simulink model "PA_Reactor_2019"  (R2018b)
settings: Solver=ode15s  StartTime=0  StopTime=400  RelTol=1e-3
libraries: simulink x13
settings Model: Creator=fmala  LastModifiedBy=andreas
settings OptimizationCC: EfficientMapNaN2IntZero=off
settings HardwareCC: TargetBitPerLong=64  TargetBitPerPointer=64  TargetBitPerSizeT=64  TargetBitPerPtrDiffT=64  TargetLongLongMode=on  TargetIntDivRoundTo=Zero  TargetEndianess=LittleEndian  TargetWordSize=64  TargetHWDeviceType=MATLAB Host  ProdEqTarget=off
settings CodeAppCC: MaxIdLength=128
settings GRTTargetCC: TargetLangStandard=C89/C90 (ANSI)  CombineOutputUpdateFcns=off  GRTInterface=on

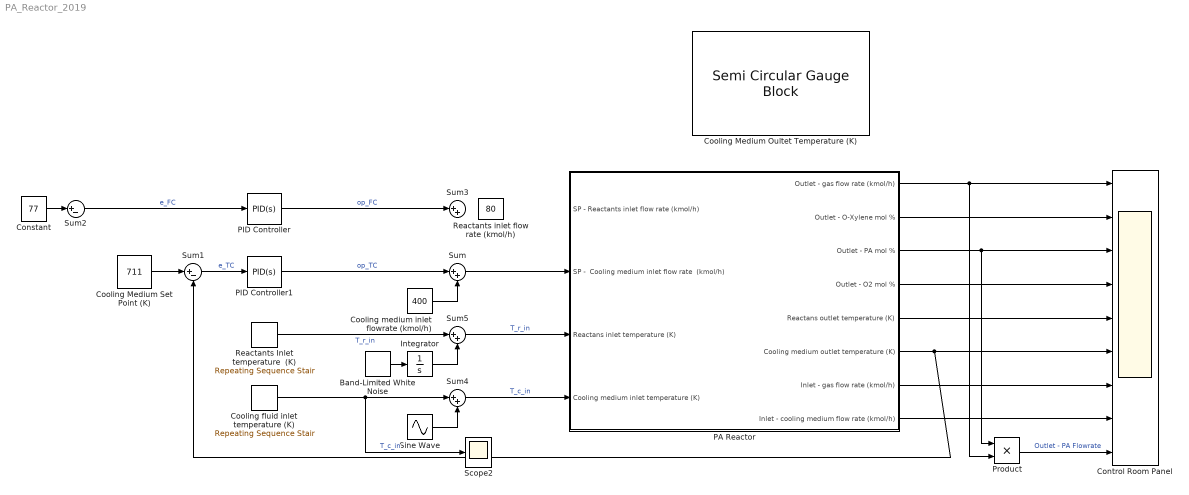
== system PA_Reactor_2019 ==
  Band-Limited White Noise : simulink/Sources/Band-Limited White Noise  Cov=1  Ts=1  seed=[23341]
  Constant : Constant  Value=77
  Control Room Panel : Scope  NumInputPorts=9
  Cooling Medium Oultet Temperature (K) : SemiCircularGaugeBlock  WebBlockId=63  ScaleMin=680  ScaleMax=780
  "Cooling Medium Set Point (K) " : Constant  Value=711  VectorParams1D=off  SampleTime=-1
  Cooling fluid inlet temperature (K) : simulink/Sources/Repeating Sequence Stair  OutValues=[680 680 685 690 695 705 705 705 705 705].'  tsamp=30  OutMin=[]  OutMax=[]  OutDataTypeStr=double  OutputDataTypeScalingMode=double  OutDataType=fixdt(0,8)  ConRadixGroup=Best Precision: Vector-wise  OutScaling=2^-12
  Cooling medium inlet flowrate (kmol/h) : Constant  Value=400
  Integrator : Integrator
  PA Reactor : Subsystem
  PID Controller : simulink/Continuous/PID Controller  Controller=PID  Form=Parallel  TimeDomain=Continuous-time  SampleTime=-1  IntegratorMethod=Forward Euler  FilterMethod=Forward Euler  ControllerParametersSource=internal  P=-0.2  I=0  D=0  UseFilter=on  N=100  TunerSelectOption=Transfer Function Based (PID Tuner App)  InitialConditionSource=internal  InitialConditionForIntegrator=0  InitialConditionForFilter=0  DifferentiatorICPrevScaledInput=0  ExternalReset=none  TrackingMode=off  Kt=1  LimitOutput=off  UpperSaturationLimit=inf  LowerSaturationLimit=-inf  LinearizeAsGain=on  AntiWindupMode=none  Kb=1  POutMin=[]  POutMax=[]  IOutMin=[]  IOutMax=[]  DOutMin=[]  DOutMax=[]  NOutMin=[]  NOutMax=[]  SumOutMin=[]  SumOutMax=[]  SaturationOutMin=[]  SaturationOutMax=[]  PParamMin=[]  PParamMax=[]  IParamMin=[]  IParamMax=[]  DParamMin=[]  DParamMax=[]  NParamMin=[]  NParamMax=[]  KbParamMin=[]  KbParamMax=[]  KtParamMin=[]  KtParamMax=[]  KbOutMin=[]  KbOutMax=[]  KtOutMin=[]  KtOutMax=[]  IntegratorOutMin=[]  IntegratorOutMax=[]  FilterOutMin=[]  FilterOutMax=[]  SumI1OutMin=[]  SumI1OutMax=[]  SumI2OutMin=[]  SumI2OutMax=[]  SumI3OutMin=[]  SumI3OutMax=[]  SumI4OutMin=[]  SumI4OutMax=[]  SumDOutMin=[]  SumDOutMax=[]  DifferentiatorOutMin=[]  DifferentiatorOutMax=[]  FilterDiffOutCoefMin=[]  FilterDiffOutCoefMax=[]  ReciprocalOutMin=[]  ReciprocalOutMax=[]  SumDenOutMin=[]  SumDenOutMax=[]  SumNumOutMin=[]  SumNumOutMax=[]  DivideOutMin=[]  DivideOutMax=[]  IntegratorContinuousStateAttributes=''  IntegratorStateMustResolveToSignalObject=off  IntegratorRTWStateStorageClass=Auto  FilterContinuousStateAttributes=''  FilterStateMustResolveToSignalObject=off  FilterRTWStateStorageClass=Auto  ParallelPVariant=InternalParameters  IdealPVariant=Disabled  IVariant=InternalParameters  DVariant=InternalParameters  IntegratorVariant=Continuous  SatVariant=Disabled  AWVariant=Passthrough  PCopyVariant=Disabled  TRVariant=Disabled  FdbkBlocksVariant=Forward  IdealPFdbkVariant=Disabled  SatFdbkVariant=Disabled  DerivativeFilterVariant=ContFilter  NVariant=InternalParameters  NCopyVariant=Disabled  FilterICVariant=InternalICsFilter  IntegratorICVariant=InternalICs  ExternalResetVariant=Disabled  TRSumVariant=Passthrough  SumFdbkVariant=Disabled  SumVariant=Sum_PID
  PID Controller1 : simulink/Continuous/PID Controller  Controller=PID  Form=Ideal  TimeDomain=Continuous-time  SampleTime=-1  IntegratorMethod=Forward Euler  FilterMethod=Forward Euler  ControllerParametersSource=internal  P=-3  I=2  D=0  UseFilter=on  N=100  TunerSelectOption=Transfer Function Based (PID Tuner App)  InitialConditionSource=internal  InitialConditionForIntegrator=0  InitialConditionForFilter=0  DifferentiatorICPrevScaledInput=0  ExternalReset=none  TrackingMode=off  Kt=1  LimitOutput=off  UpperSaturationLimit=inf  LowerSaturationLimit=-inf  LinearizeAsGain=on  AntiWindupMode=none  Kb=1  POutMin=[]  POutMax=[]  IOutMin=[]  IOutMax=[]  DOutMin=[]  DOutMax=[]  NOutMin=[]  NOutMax=[]  SumOutMin=[]  SumOutMax=[]  SaturationOutMin=[]  SaturationOutMax=[]  PParamMin=[]  PParamMax=[]  IParamMin=[]  IParamMax=[]  DParamMin=[]  DParamMax=[]  NParamMin=[]  NParamMax=[]  KbParamMin=[]  KbParamMax=[]  KtParamMin=[]  KtParamMax=[]  KbOutMin=[]  KbOutMax=[]  KtOutMin=[]  KtOutMax=[]  IntegratorOutMin=[]  IntegratorOutMax=[]  FilterOutMin=[]  FilterOutMax=[]  SumI1OutMin=[]  SumI1OutMax=[]  SumI2OutMin=[]  SumI2OutMax=[]  SumI3OutMin=[]  SumI3OutMax=[]  SumI4OutMin=[]  SumI4OutMax=[]  SumDOutMin=[]  SumDOutMax=[]  DifferentiatorOutMin=[]  DifferentiatorOutMax=[]  FilterDiffOutCoefMin=[]  FilterDiffOutCoefMax=[]  ReciprocalOutMin=[]  ReciprocalOutMax=[]  SumDenOutMin=[]  SumDenOutMax=[]  SumNumOutMin=[]  SumNumOutMax=[]  DivideOutMin=[]  DivideOutMax=[]  IntegratorContinuousStateAttributes=''  IntegratorStateMustResolveToSignalObject=off  IntegratorRTWStateStorageClass=Auto  FilterContinuousStateAttributes=''  FilterStateMustResolveToSignalObject=off  FilterRTWStateStorageClass=Auto  ParallelPVariant=Passthrough  IdealPVariant=InternalParameters  IVariant=InternalParameters  DVariant=InternalParameters  IntegratorVariant=Continuous  SatVariant=Disabled  AWVariant=Passthrough  PCopyVariant=Disabled  TRVariant=Disabled  FdbkBlocksVariant=Forward  IdealPFdbkVariant=Disabled  SatFdbkVariant=Disabled  DerivativeFilterVariant=ContFilter  NVariant=InternalParameters  NCopyVariant=Disabled  FilterICVariant=InternalICsFilter  IntegratorICVariant=InternalICs  ExternalResetVariant=Disabled  TRSumVariant=Passthrough  SumFdbkVariant=Disabled  SumVariant=Sum_PID
  Product : Product
  Reactants Inlet temperature  (K) : simulink/Sources/Repeating Sequence Stair  OutValues=[690].'  tsamp=10  OutMin=[]  OutMax=[]  OutDataTypeStr=double  OutputDataTypeScalingMode=double  OutDataType=fixdt(0,8)  ConRadixGroup=Best Precision: Vector-wise  OutScaling=2^-12
  "Reactants inlet flow rate (kmol/h) " : Constant  Value=80
  Scope2 : Scope
  Sine Wave : Sin  Amplitude=20  Frequency=pi/200  SampleTime=0
  Sum{,3..5} (4 alike) : Sum  Inputs=|++
  Sum1 : Sum  Inputs=|+-
  Sum2 : Sum  Inputs=|+-
  wires:
  PA Reactor/1(Outlet - gas flow rate (kmol/h)) -> Control Room Panel/1, Product/2
  PA Reactor/2(Outlet - O-Xylene mol %) -> Control Room Panel/2
  PA Reactor/3(Outlet - PA mol %) -> Control Room Panel/3, Product/1
  PA Reactor/4(Outlet - O2 mol %) -> Control Room Panel/4
  PA Reactor/7(Inlet - gas flow rate (kmol/h)) -> Control Room Panel/7
  PA Reactor/8(Inlet - cooling medium flow rate (kmol/h)) -> Control Room Panel/8
  PA Reactor/6(Cooling medium outlet temperature (K)) -> Sum1/2, Control Room Panel/6
  Cooling fluid inlet temperature (K)/1 -> Sum4/1, Scope2/1  "T_c_in"
  Sum1/1 -> PID Controller1/1  "e_TC"
  PID Controller1/1 -> Sum/1  "op_TC"
  PA Reactor/5(Reactans outlet temperature (K)) -> Control Room Panel/5
  Constant/1 -> Sum2/1
  Sum2/1 -> PID Controller/1  "e_FC"
  PID Controller/1 -> Sum3/1  "op_FC"
  Cooling medium inlet flowrate (kmol/h)/1 -> Sum/2
  Sum/1 -> PA Reactor/2(SP -  Cooling medium inlet flow rate  (kmol/h))
  "Cooling Medium Set Point (K) "/1 -> Sum1/1
  Sum4/1 -> PA Reactor/4(Cooling medium inlet temperature (K))  "T_c_in"
  Sine Wave/1 -> Sum4/2
  Reactants Inlet temperature  (K)/1 -> Sum5/1  "T_r_in"
  Sum5/1 -> PA Reactor/3(Reactans inlet temperature (K))  "T_r_in"
  Integrator/1 -> Sum5/2
  Band-Limited White Noise/1 -> Integrator/1
  Product/1 -> Control Room Panel/9  "Outlet - PA Flowrate"

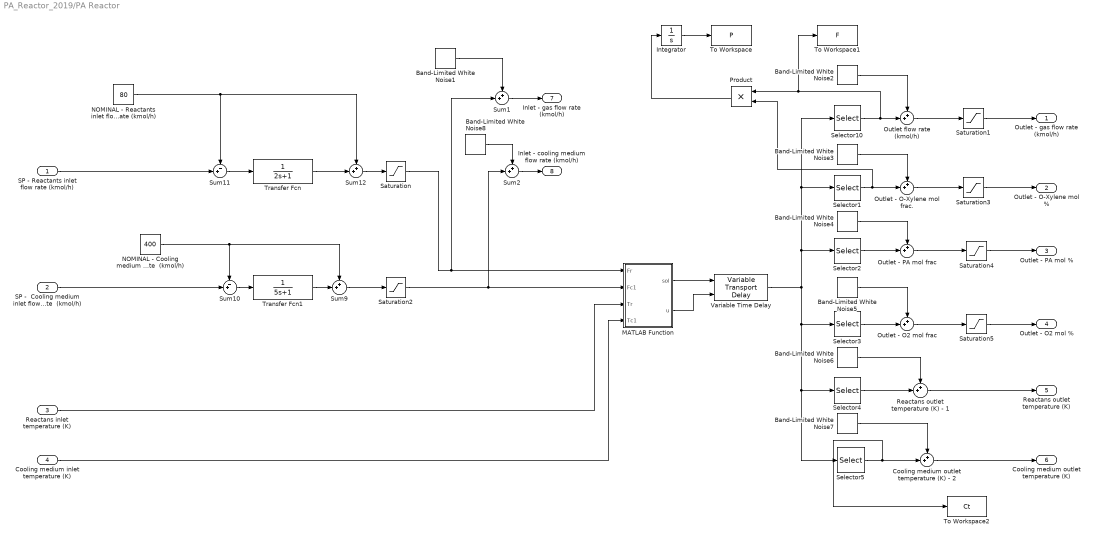
== system PA_Reactor_2019/PA Reactor ==
  SP - Reactants inlet flow rate (kmol/h) : Inport
  SP -  Cooling medium inlet flow rate  (kmol/h) : Inport  Port=2
  Reactans inlet temperature (K) : Inport  Port=3
  Cooling medium inlet temperature (K) : Inport  Port=4
  Band-Limited White Noise1 : simulink/Sources/Band-Limited White Noise  Cov=[0.001]  Ts=0.01  seed=[1111]
  Band-Limited White Noise2 : simulink/Sources/Band-Limited White Noise  Cov=[0.001]  Ts=0.01  seed=[1]
  Band-Limited White Noise3 : simulink/Sources/Band-Limited White Noise  Cov=[0.0001]  Ts=0.5  seed=[3341]
  Band-Limited White Noise4 : simulink/Sources/Band-Limited White Noise  Cov=[0.0001]  Ts=0.5  seed=[2355341]
  Band-Limited White Noise5 : simulink/Sources/Band-Limited White Noise  Cov=[0.0001]  Ts=0.5  seed=[7341]
  Band-Limited White Noise6 : simulink/Sources/Band-Limited White Noise  Cov=[0.002]  Ts=0.01  seed=[241]
  Band-Limited White Noise7 : simulink/Sources/Band-Limited White Noise  Cov=[0.008]  Ts=0.03  seed=[23341]
  Band-Limited White Noise8 : simulink/Sources/Band-Limited White Noise  Cov=[0.001]  Ts=0.01  seed=[1575777]
  Cooling medium outlet temperature (K) - 2 : Sum  Inputs=++|
  Integrator : Integrator
  MATLAB Function : MATLAB Function  TreatAsAtomicUnit=on
  NOMINAL - Cooling medium inlet flow rate  (kmol/h) : Constant  Value=400
  NOMINAL - Reactants inlet flow rate (kmol/h) : Constant  Value=80
  Outlet - O-Xylene mol frac. : Sum  Inputs=++|
  Outlet - O2 mol frac : Sum  Inputs=++|
  Outlet - PA mol frac : Sum  Inputs=++|
  Outlet flow rate (kmol/h) : Sum  Inputs=++|
  Product : Product
  Reactans outlet temperature (K) - 1 : Sum  Inputs=++|
  Saturation : Saturate  UpperLimit=250  LowerLimit=10
  Saturation1 : Saturate  UpperLimit=500  LowerLimit=0
  Saturation2 : Saturate  UpperLimit=1000  LowerLimit=100
  Saturation3 : Saturate  UpperLimit=100  LowerLimit=0
  Saturation4 : Saturate  UpperLimit=100  LowerLimit=0
  Saturation5 : Saturate  UpperLimit=100  LowerLimit=0
  Selector1 : Selector  InputPortWidth=6  IndexOptions=Index vector (dialog)  Indices=[2]  OutputSizes=1
  Selector10 : Selector  InputPortWidth=6  IndexOptions=Index vector (dialog)  Indices=[1]  OutputSizes=1
  Selector2 : Selector  InputPortWidth=6  IndexOptions=Index vector (dialog)  Indices=[3]  OutputSizes=1
  Selector3 : Selector  InputPortWidth=6  IndexOptions=Index vector (dialog)  Indices=[4]  OutputSizes=1
  Selector4 : Selector  InputPortWidth=6  IndexOptions=Index vector (dialog)  Indices=[5]  OutputSizes=1
  Selector5 : Selector  InputPortWidth=6  IndexOptions=Index vector (dialog)  Indices=[6]  OutputSizes=1
  Sum{1..2,9,12} (4 alike) : Sum  Inputs=++|
  Sum10 : Sum  Inputs=-+|
  Sum11 : Sum  Inputs=-+|
  To Workspace : ToWorkspace  VariableName=P  SaveFormat=Timeseries  SampleTime=-1
  To Workspace1 : ToWorkspace  VariableName=F  SaveFormat=Timeseries  SampleTime=-1
  To Workspace2 : ToWorkspace  VariableName=Ct  SaveFormat=Timeseries  SampleTime=-1
  Transfer Fcn : TransferFcn  Denominator=[2 1]
  Transfer Fcn1 : TransferFcn  Denominator=[5 1]
  Variable Time Delay : VariableTransportDelay  MaximumDelay=25  InitialOutput=[90.36 0 0.85 2.12 711 711]  MaximumPoints=3072  ZeroDelay=on
  Outlet - gas flow rate (kmol/h) : Outport
  Outlet - O-Xylene mol % : Outport  Port=2
  Outlet - PA mol % : Outport  Port=3
  Outlet - O2 mol % : Outport  Port=4
  Reactans outlet temperature (K) : Outport  Port=5
  Cooling medium outlet temperature (K) : Outport  Port=6
  Inlet - gas flow rate (kmol/h) : Outport  Port=7
  Inlet - cooling medium flow rate (kmol/h) : Outport  Port=8
  wires:
  Selector3/1 -> Outlet - O2 mol frac/2
  Variable Time Delay/1 -> Selector1/1, Selector10/1, Selector2/1, Selector5/1, Selector4/1, Selector3/1
  NOMINAL - Cooling medium inlet flow rate  (kmol/h)/1 -> Sum9/1, Sum10/1
  Band-Limited White Noise4/1 -> Outlet - PA mol frac/1
  Sum10/1 -> Transfer Fcn1/1
  MATLAB Function/1(sol) -> Variable Time Delay/1
  Band-Limited White Noise2/1 -> Outlet flow rate (kmol/h)/1
  Selector10/1 -> Outlet flow rate (kmol/h)/2, To Workspace1/1, Product/1
  Selector1/1 -> Outlet - O-Xylene mol frac./2, Product/2
  Reactans inlet temperature (K)/1 -> MATLAB Function/3(Tr)
  Band-Limited White Noise6/1 -> Reactans outlet temperature (K) - 1/1
  Sum9/1 -> Saturation2/1
  Sum12/1 -> Saturation/1
  Outlet - O-Xylene mol frac./1 -> Saturation3/1
  Outlet - PA mol frac/1 -> Saturation4/1
  MATLAB Function/2(u) -> Variable Time Delay/2
  Selector2/1 -> Outlet - PA mol frac/2
  Selector4/1 -> Reactans outlet temperature (K) - 1/2
  Band-Limited White Noise3/1 -> Outlet - O-Xylene mol frac./1
  Band-Limited White Noise7/1 -> Cooling medium outlet temperature (K) - 2/1
  Cooling medium inlet temperature (K)/1 -> MATLAB Function/4(Tc1)
  Saturation/1 -> Sum1/2, MATLAB Function/1(Fr)
  Transfer Fcn/1 -> Sum12/2
  Transfer Fcn1/1 -> Sum9/2
  Saturation2/1 -> MATLAB Function/2(Fc1), Sum2/2
  Outlet flow rate (kmol/h)/1 -> Saturation1/1
  NOMINAL - Reactants inlet flow rate (kmol/h)/1 -> Sum12/1, Sum11/1
  Reactans outlet temperature (K) - 1/1 -> Reactans outlet temperature (K)/1
  Band-Limited White Noise5/1 -> Outlet - O2 mol frac/1
  SP - Reactants inlet flow rate (kmol/h)/1 -> Sum11/2
  Sum11/1 -> Transfer Fcn/1
  Product/1 -> Integrator/1
  Cooling medium outlet temperature (K) - 2/1 -> Cooling medium outlet temperature (K)/1
  SP -  Cooling medium inlet flow rate  (kmol/h)/1 -> Sum10/2
  Selector5/1 -> To Workspace2/1, Cooling medium outlet temperature (K) - 2/2
  Outlet - O2 mol frac/1 -> Saturation5/1
  Band-Limited White Noise1/1 -> Sum1/1
  Band-Limited White Noise8/1 -> Sum2/1
  Sum2/1 -> Inlet - cooling medium flow rate (kmol/h)/1
  Sum1/1 -> Inlet - gas flow rate (kmol/h)/1
  Saturation1/1 -> Outlet - gas flow rate (kmol/h)/1
  Saturation3/1 -> Outlet - O-Xylene mol %/1
  Saturation4/1 -> Outlet - PA mol %/1
  Saturation5/1 -> Outlet - O2 mol %/1
  Integrator/1 -> To Workspace/1

== matlab function PA_Reactor_2019/PA Reactor/MATLAB Function ==
  data: Fr input; sol output; u output; Fc1 input; Tr input; Tc1 input
function [sol,u]= fcn(Fr, Fc1, Tr, Tc1)

Data_c = [24.99735 55.18696 -33.69137 7.948387 -0.136638 106.16; %O-Xylene  // Order is (1-5) A B C D E for Cp calculation (6) MW
        24.99735 55.18696 -33.69137 7.948387 -0.136638 148.1; %Phthalic anhydride
        24.99735 55.18696 -33.69137 7.948387 -0.136638 44.0095  % Carbon dioxide
        25.56759 6.096130 4.054656  -2.67130 0.131021  28.0101; % Carbon monoxide
        30.09200 6.832514 6.793435 -2.534480 0.082139  18.0153; % Water
        23.4333  21.3322  -13.5029  3.5781   0         31.9988; % Oxygen
        19.50583 19.88705 -8.598535 1.369784 0.527601  28.0134]; % Nitrogen

f1 = 0.2;
    
Data_r = [-1283000 * f1 -1526200 * f1 -3273600 * f1 -265600 * f1 -1398000 * f1;  % Enthalpy of Reaction[kJ/kmol] // Order: Reaction 1-5
          19.84*1.143    20.34     20.86   18.34   19.51;     %Ln k0
          13636    14394     14394   15803   15803];    %E/R [K]  
      
Constant = [8.314459848e-2        %(1) R [m3 Bar K-1 kmol-1] 
            9.80665               %(2) g m/s^2
            .8                    %(3) d Reactor inner diameter m
            .8^2 * 3.1416 / 4     %(4) Reactor Area m^2
            20                    %(5) Reactor length m
            0.282                 %(6) n
            429                   %(7) b1 bar-1 
            2024                  %(8) b2 bar-1
            8                     %(9) Initial Pressure bar 
            0.4                   %(10) bed voidage  
            7.04 / 1000           %(11) equivalent particle diameter m  
            0.45                  %(12) U kW/m2K 
            7.5];                   %(13) Cp kJ/kmol.K                                

CompNot = [1.5 0 0 0 0 20 80]; % Composition Mol Frac / not normalized (1) O-Xylene (2) Phthalic anhydride (3) Carbon dioxide (4) Carbon monoxide (5) Water % (6)Oxygen (7) Nitrogen
Comp = CompNot/sum(CompNot); % Composition Mol Frac (1) O-Xylene (2) Phthalic anhydride (3) Carbon dioxide (4) Carbon monoxide (5) Water % (6)Oxygen (7) Nitrogen
           
Fr = Fr / 3600;     %Flow kmol/s
Fc1 = Fc1 /1000;      %Flow kmol/s

Ini = [Fr * Comp Fc1 Tr Tc1 Constant(9)];
zspan = 0:Constant(5)/50:Constant(5);
[z,y] = ode23(@(z,y) reactor(z, y, Constant, Data_r, Data_c), zspan, Ini);

F_f = (y(end,1)+y(end,2)+y(end,3)+y(end,4)+y(end,5)+y(end,6)+y(end,7));
PA_f = y(end,2)/F_f*100;
OX_f = y(end,1)/F_f*100;
O2_f = y(end,6)/F_f*100;
F_f = (y(end,1)+y(end,2)+y(end,3)+y(end,4)+y(end,5)+y(end,6)+y(end,7)) * 3600;
Tc_f = y(end,10);
Tr_f = y(end,9);

Vel = Fr * Constant(1) * Tr / Constant(9) / Constant(4); %m/s
u = Constant(5) / Vel / 4 ; %s
sol = [F_f, OX_f, PA_f, O2_f, Tr_f, Tc_f]'; 
sol(sol<0) = 0; %All the values compositions, and absolute temepratures and pressures have to be positive

function diff = reactor(z, y, Constant, Data_r, Data_c)

n = Constant(6);
D = Constant(3);
R = Constant(1);
A = Constant(4);
b1 = Constant(7); 
b2 = Constant(8);
e = Constant(10);
Dp = Constant(11);
U = Constant(12);
Cp = Constant(13); 

y(y<0) = 0; %All the values compositions, and absolute temepratures and pressures have to be positive

Fc = y(8);
T = y(9);
Tc = y(10);
P = y(11);

Xyl = y(1); % Flowrate calculations kmol/s
Pht = y(2);
CO2 = y(3);
CO  = y(4);
H2O = y(5);
O2  = y(6);
N2  = y(7);

F = Xyl + Pht + CO2 + CO + H2O + O2 + N2; %molar flow kmol/s
M = Xyl * Data_c(1,6) + Pht * Data_c(2,6) + CO2 * Data_c(3,6) + CO * Data_c(4,6) + H2O * Data_c(5,6) + O2 * Data_c(6,6) + N2 * Data_c(7,6); %mass flow kg/s
V = F * R * T / P; %volume flow m3/s
rho = M / V; %density kg/m3

pXyl = P * y(1) / F; %bar
pPht = P * y(2) / F;
pO2  = P * y(6) / F; 

r1 = kj(T,1,Data_r) * pO2^n * b1 * pXyl / (1 + b1 * pXyl);    %[kg / h m3]
r2 = kj(T,2,Data_r) * pO2^n * b2 * pXyl / (1 + b2 * pXyl);    
r3 = kj(T,3,Data_r) * pO2^n * b2 * pXyl / (1 + b2 * pXyl);    
r4 = kj(T,4,Data_r) * pO2^n * pPht;      
r5 = kj(T,5,Data_r) * pO2^n * pPht;       

dXyldz = (-r1 - r2 - r3) * A / Data_c(1,6) / 3600;   %[kmol/s.m]
dPhtdz = (r1 - r4 - r5)  * A / Data_c(2,6) / 3600;
dCO2dz = 8 * (r3 + r5)   * A / Data_c(3,6) / 3600;
dCOdz =  8 * (r2 + r4)    * A / Data_c(4,6) / 3600; 
dH2Odz = ( 3 * r1 + 5 * (r2 + r3) + 2 * (r4 + r5)) * A / Data_c(5,6) / 3600;
dO2dz = (-3 * r1 - 6.5 * r2 - 10.5 * r3 - 4.5 * r4 - 7.5 * r5 ) * A / Data_c(6,6) / 3600; 
dN2dz = 0 / Data_c(7,6) / 3600;

dFcdz = 0; %no change in the flowrate of coolant

DTML = (Tc - T);
dQc = U * (Fc)^0.5 * D * 3.14 * DTML; 
dTcdz =  - dQc / (Cp * Fc);

dTrdz = -((r1 * Data_r(1,1) / Data_c(1,6) + r2 * Data_r(1,2) / Data_c(2,6) + r3 * Data_r(1,3) / Data_c(3,6) + r4 * Data_r(1,4) / Data_c(4,6) + r5 * Data_r(1,5) / Data_c(5,6))  *  A / 3600 - dQc )/... 
        (Xyl * HeatCap(1,T,Data_c) + O2 * HeatCap(6,T,Data_c) + N2 * HeatCap(7,T,Data_c) + CO * HeatCap(4,T,Data_c) + CO2 * HeatCap(3,T,Data_c) + Pht * HeatCap(2,T,Data_c) + H2O * HeatCap(5,T,Data_c));

dPdz =  -1.75 *(M/A)^2 * (1-e) / (Dp * rho * e^3) / 10^5; %bar/m
diff = [dXyldz dPhtdz dCO2dz dCOdz dH2Odz dO2dz dN2dz dFcdz dTrdz dTcdz dPdz]';
end

function KJ = kj(T,n,R) % rate contant calculation [(kmol/m3)1-n/s] n=0.282 
  KJ = exp(R(2,n)-R(3,n)/T); 
end

function Cp = HeatCap(C,T,Chem) %Gas Phase Heat Capacity (Shomate Equation) // Cp = heat capacity (J/mol*K)
    Cp = Chem(C,1) + Chem(C,2) * T/1000 + Chem(C,3) * ( T / 1000)^2 + Chem(C,4) * ( T / 1000)^3 + Chem(C,5) / (( T / 1000)^2);
end
end
